simulink model "observer_theory"  (R2024b)
settings: Solver=VariableStepAuto  StartTime=0.0  StopTime=20  MaxStep=0.1  RelTol=1e-3
undefined symbols (not defined in the file or in its folder): beta0, J, K, R, r
libraries: cstblocks x1
settings Model: Creator=icpmoles  LastModifiedBy=icpmoles

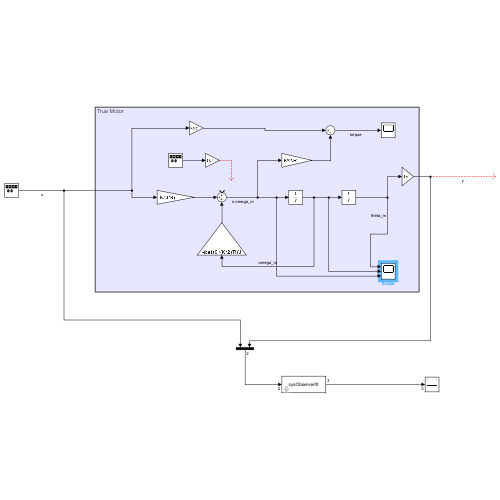
[thumbnail: Simulink's stored preview of the top-level diagram]
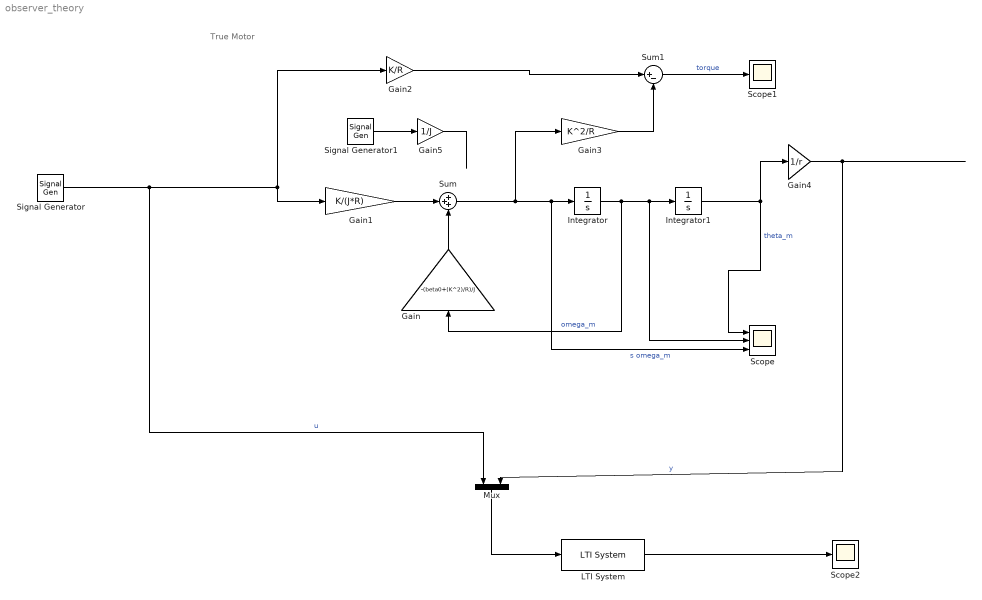
== system observer_theory ==
  note: True Motor
  Gain : Gain  Gain=-(beta0+(K^2)/R)/J
  Gain1 : Gain  Gain=K/(J*R)
  Gain2 : Gain  Gain=K/R
  Gain3 : Gain  Gain=K^2/R
  Gain4 : Gain  Gain=1/r
  Gain5 : Gain  Gain=1/J
  Integrator : Integrator
  Integrator1 : Integrator
  LTI System : cstblocks/LTI System  sys=sysObserver0t  IC=[]  PadeOrder=0
  Mux : Mux  Inputs=2
  Scope : Scope  NumInputPorts=3
  Scope1 : Scope
  Scope2 : Scope
  Signal Generator : SignalGenerator  Frequency=3  Units=rad/sec
  Signal Generator1 : SignalGenerator  Amplitude=0.001  Frequency=0.1  Units=rad/sec
  Sum : Sum  Inputs=+++
  Sum1 : Sum  Inputs=|+-
  wires:
  Integrator/1 -> Gain/1, Scope/2, Integrator1/1  "omega_m"
  Signal Generator/1 -> Mux/1, Gain1/1, Gain2/1  "u"
  Gain/1 -> Sum/3
  Gain1/1 -> Sum/2
  Sum/1 -> Gain3/1, Integrator/1, Scope/3  "s omega_m"
  Gain2/1 -> Sum1/1
  Gain3/1 -> Sum1/2
  Sum1/1 -> Scope1/1  "torque"
  Integrator1/1 -> Gain4/1, Scope/1  "theta_m"
  Gain4/1 -> Mux/2  "y"
  Mux/1 -> LTI System/1
  LTI System/1 -> Scope2/1
  Gain5/1 -> ?
  Signal Generator1/1 -> Gain5/1
